simulink model "UnitDelay"  (R2015b)
settings: Solver=VariableStepAuto  StartTime=0.0  StopTime=10.0  RelTol=1e-3
settings Model: Creator=LUBO  LastModifiedBy=LUBO

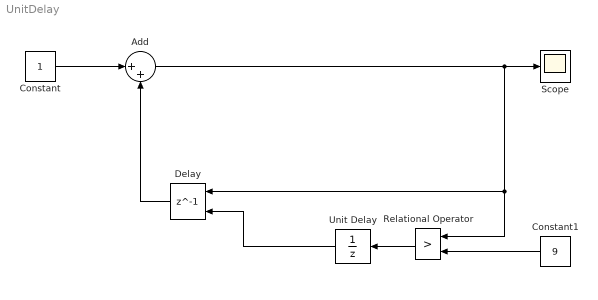
== system UnitDelay ==
  Add : Sum  Inputs=|++
  Constant : Constant
  Constant1 : Constant  Value=9
  Delay : Delay  DelayLength=1  InitialCondition=0  ExternalReset=Rising
      settings: InputPortMap=u0,r5
  Relational Operator : RelationalOperator  Operator=>  OutDataTypeStr=boolean
  Scope : Scope
  Unit Delay : UnitDelay  SampleTime=0.5
  wires:
  Constant1/1 -> Relational Operator/2
  Relational Operator/1 -> Unit Delay/1
  Unit Delay/1 -> Delay/2
  Constant/1 -> Add/1
  Delay/1 -> Add/2
  Add/1 -> Delay/1, Relational Operator/1, Scope/1
